simulink model "Ex2"  (R2023a)
settings: Solver=VariableStepAuto  StartTime=0.0  StopTime=3  RelTol=1e-3
settings Model: Creator=gutoc  LastModifiedBy=gutoc

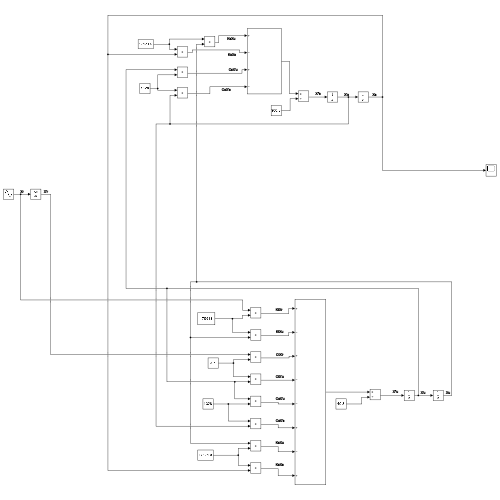
[thumbnail: Simulink's stored preview of the top-level diagram]
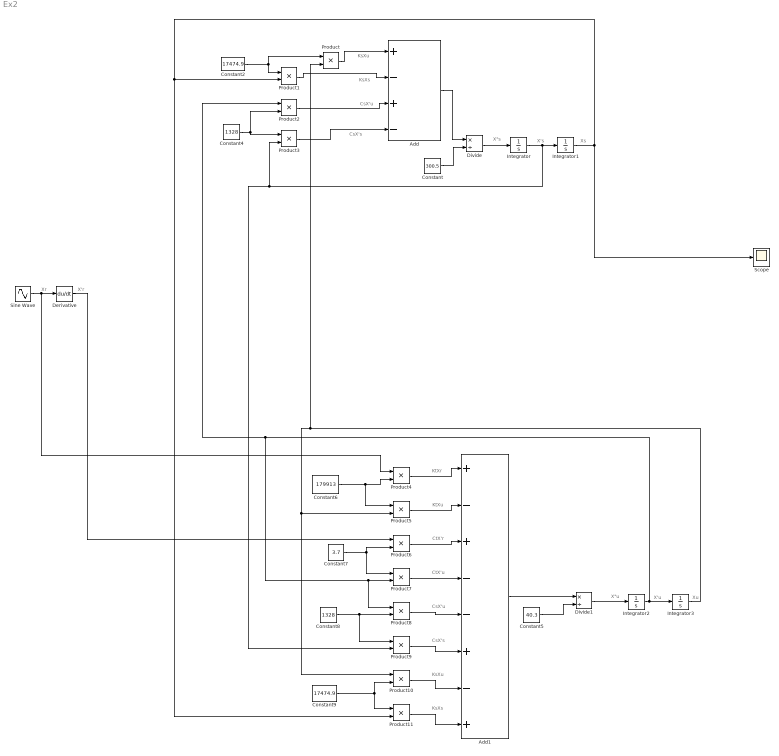
== system Ex2 ==
  note: KsXs
  note: Xr
  note: Xs
  note: X'u
  note: X"u
  note: X's
  note: X"s
  note: X'r
  note: Xu
  note: KsXu
  note: CsX'u
  note: CsX's
  note: KtXr
  note: KtXu
  note: CtX'r
  note: CtX'u
  note: CsX'u
  note: CsX's
  note: KsXu
  note: KsXs
  Add : Sum  Inputs=+-+-
  Add1 : Sum  Inputs=+-+--+-+
  Constant : Constant  Value=300.5
  Constant2 : Constant  Value=17474.9
  Constant4 : Constant  Value=1328
  Constant5 : Constant  Value=40.3
  Constant6 : Constant  Value=179913
  Constant7 : Constant  Value=3.7
  Constant8 : Constant  Value=1328
  Constant9 : Constant  Value=17474.9
  Derivative : Derivative
  Divide : Product  Inputs=*/
  Divide1 : Product  Inputs=*/
  Integrator{,1..3} (4 alike) : Integrator
  Product{,1..11} (12 alike) : Product
  Scope : Scope
  Sine Wave : Sin  Amplitude=0.001  Bias=0.01  SampleTime=0
  wires:
  Derivative/1 -> Product6/1
  Product4/1 -> Add1/1
  Divide1/1 -> Integrator2/1
  Constant7/1 -> Product6/2, Product7/1
  Product8/1 -> Add1/5
  Integrator2/1 -> Product2/1, Product8/1, Product7/2, Integrator3/1
  Product6/1 -> Add1/3
  Constant9/1 -> Product11/1, Product10/2
  Product5/1 -> Add1/2
  Constant6/1 -> Product5/1, Product4/2
  Product9/1 -> Add1/6
  Product7/1 -> Add1/4
  Constant5/1 -> Divide1/2
  Product11/1 -> Add1/8
  Product3/1 -> Add/4
  Product1/1 -> Add/2
  Constant/1 -> Divide/2
  Add/1 -> Divide/1
  Add1/1 -> Divide1/1
  Sine Wave/1 -> Derivative/1, Product4/1
  Product/1 -> Add/1
  Product2/1 -> Add/3
  Product10/1 -> Add1/7
  Constant4/1 -> Product2/2, Product3/1
  Constant8/1 -> Product9/1, Product8/2
  Constant2/1 -> Product/1, Product1/1
  Divide/1 -> Integrator/1
  Integrator1/1 -> Product11/2, Product1/2, Scope/1
  Integrator3/1 -> Product/2, Product10/1, Product5/2
  Integrator/1 -> Product9/2, Product3/2, Integrator1/1
